simulink model "main_RI_LIEKF"  (R2023a)
settings: Solver=FixedStepAuto  StartTime=0.0  StopTime=220  FixedStep=0.01  RelTol=1e-3
InitFcn:
  | initNavigation0612_AOA;
values from neighbouring files (symbols this model uses):
  CF_enable = 0    [initNavigation.m]
  dt = 0.01    [initNavigation.m]
  dtDelay = -0.03    [initNavigation.m]
  g0 = 9.795    [initNavigation.m]
  gam0_rad = 0/57.3    (= 0)    [initNavigation.m]
  H_sensor_type = 0    [initNavigation.m]
  KF_enable = 1    [initNavigation.m]
  P0 = diag([1*ones(3,1);0.01*ones(3,1);0.1*ones(3,1);0.001*ones(3,1);0.00001*ones(3,1)])    [initNavigation.m]
  P0_RIEKF = diag([1*ones(3,1);0.01*ones(3,1);0.1*ones(3,1);0.001*ones(3,1);0.00001*ones(3,1);      0.01*ones(3,1);[0;2;2]/57.3;[0.1;0.1;0.1]])^2    [initNavigation.m]
  pd0 = 0    [initNavigation.m]
  pe0 = 0    [initNavigation.m]
  phi0_rad = 0/57.3    (= 0)    [initNavigation.m]
  pn0 = 0    [initNavigation.m]
  psi = -178    [initNavigation.m]
  psi0_rad = 0/57.3    (= 0)    [initNavigation.m]
  state_dim = 24    [initNavigation.m]
  Time = 0:0.01:(size(traindata.AttackAngle,1) - 1)*0.01    [NNLiftCoefficientFit.m]
  vd0 = 0    [initNavigation.m]
  ve0 = 0    [initNavigation.m]
  vn0 = 0    [initNavigation.m]
undefined symbols (not defined in the file or in its folder): DiscIntNeverNeededParam, Discrete, INS_CONST, INS_EXPORT, INS_PARAM, magnitude, p, param, pInitialization, sys
libraries: simulink x69, simulink_extras x64, dspstat3 x56, sharedtransform x49, ctrlSharedLib x36, sharedTrackingLibrary x17, FMT_Model_Lib x13, matrix_library x12, deeplib x4, dspsolvers x4, vrlib x4, aerolibconvert2 x1
(part 15 of 22)

== system main_RI_LIEKF/State estimation/bak1/INS propogation/Init_PVQ/Horizontal_attitude ==
  note: gamma
  note: fai
  accl_mean_B_m/s_LPF : Inport  PortDimensions=3
  Magn_mean_B_guess_LPF : Inport  Port=2
  Enable : EnablePort
  Add : Sum  Inputs=+-
  Asin : Trigonometry  Operator=asin
  Atan2 : Trigonometry  Operator=atan2
  Data Type Conversion : DataTypeConversion  SaturateOnIntegerOverflow=off  RndMeth=Floor
  Deal with zero : Subsystem
  Degrees to Radians : simulink_extras/Transformations/Degrees to Radians
  Degrees to Radians1 : simulink_extras/Transformations/Degrees to Radians
  Demux : Demux  Outputs=3
  Divide : Product  Inputs=*/  OutDataTypeStr=single
  Gain1 : Gain  Gain=-1
  Gain2 : Gain  Gain=-1
  Magnetic declination : Constant  Value=param.fusion.magDeclDeg  OutDataTypeStr=single
  Magnetic declination1 : Constant  Value=param.control.MagnheadingCorrection  OutDataTypeStr=uint8
  Math Function : Math  Operator=magnitude^2  SignedPower=on
  Mux : Mux  Inputs=3
  Mux1 : Mux  Inputs=3
  Mux3 : Mux  Inputs=3
  Product : Product  Multiplication=Matrix(*)
  Quaternions to Direction Cosine Matrix : sharedtransform/Quaternions to  Direction Cosine Matrix  aMode=aMode
  Rotation Angles to Quaternions : sharedtransform/Rotation Angles to Quaternions  rotationOrder=ZYX  aMode=aMode
  Rotation Angles to Quaternions1 : sharedtransform/Rotation Angles to Quaternions  rotationOrder=ZYX  aMode=aMode
  Scope : Scope
  Scope1 : Scope
  Selector : Selector  InputPortWidth=3  IndexOptions=Index vector (dialog)  Indices=[2]  OutputSizes=1
  Selector1 : Selector  InputPortWidth=3  IndexOptions=Index vector (dialog)  Indices=[1]  OutputSizes=1
  Sqrt : Sqrt
  Sum of Elements : Sum  Inputs=+
  Switch : Switch  Threshold=0.5  SaturateOnIntegerOverflow=off  InputSameDT=off
  Terminator : Terminator
  Transpose : Math  Operator=transpose  SignedPower=on
  Trigonometric Function1 : Trigonometry  Operator=atan2
  psi_zero : Constant  Value=psi  OutDataTypeStr=single
  quat_0 : Outport  PortDimensions=4
  wires:
  Data Type Conversion/1 -> Scope/1
  Switch/1 -> quat_0/1, Scope1/1
  Magnetic declination1/1 -> Switch/2, Data Type Conversion/1
  Degrees to Radians/1 -> Terminator/1
  Degrees to Radians1/1 -> Mux1/1
  Gain1/1 -> Mux/3, Trigonometric Function1/2
  Transpose/1 -> Product/1
  Mux3/1 -> Rotation Angles to Quaternions1/1
  Add/1 -> Mux3/1  "psi_calbymag"
  Magnetic declination/1 -> Degrees to Radians/1
  Atan2/1 -> Add/2
  Selector/1 -> Atan2/1  "magE"
  Selector1/1 -> Atan2/2  "magN"
  Product/1 -> Selector1/1, Selector/1  "magNED"
  Magn_mean_B_guess_LPF/1 -> Product/2
  Quaternions to Direction Cosine Matrix/1 -> Transpose/1
  Rotation Angles to Quaternions/1 -> Quaternions to Direction Cosine Matrix/1, Switch/3  "q0_no_yaw"
  Gain2/1 -> Mux1/3, Mux3/3
  Asin/1 -> Mux1/2, Mux3/2
  psi_zero/1 -> Degrees to Radians1/1
  Mux1/1 -> Rotation Angles to Quaternions/1
  Math Function/1 -> Sum of Elements/1
  Mux/1 -> Math Function/1
  Divide/1 -> Asin/1
  Sum of Elements/1 -> Sqrt/1
  Demux/3 -> Gain1/1
  Demux/2 -> Trigonometric Function1/1, Mux/1
  Demux/1 -> Mux/2, Divide/1
  Trigonometric Function1/1 -> Gain2/1
  Deal with zero/1(Out1) -> Divide/2
  Sqrt/1 -> Deal with zero/1(In1)
  accl_mean_B_m/s_LPF/1 -> Demux/1
  Rotation Angles to Quaternions1/1 -> Switch/1

== system main_RI_LIEKF/State estimation/bak1/INS propogation/Init_PVQ/Subsystem ==
  data : Inport
  Buffer : Buffer  N=50  V=49  OutputFrames=off
  Buffer1 : Buffer  N=50  V=49  OutputFrames=off
  Buffer2 : Buffer  N=50  V=49  ic=-g0  OutputFrames=off
  Demux : Demux  Outputs=3
  Mean4 : dspstat3/Mean  run=off  reset_popup=None  directionMode=Entire input  dimension=3  roiEnable=off  roiType=Rectangles  roiPortion=Entire ROI  roiOutput=Individual statistics for each ROI  roiFlag=off  roundingMode=Floor  overflowMode=off  outputDataTypeStr=Inherit: Same as accumulator  outputMin=[]  outputMax=[]  outputLastDataTypeStr=Inherit: Same as accumulator
  Mean5 : dspstat3/Mean  run=off  reset_popup=None  directionMode=Entire input  dimension=3  roiEnable=off  roiType=Rectangles  roiPortion=Entire ROI  roiOutput=Individual statistics for each ROI  roiFlag=off  roundingMode=Floor  overflowMode=off  outputDataTypeStr=Inherit: Same as accumulator  outputMin=[]  outputMax=[]  outputLastDataTypeStr=Inherit: Same as accumulator
  Mean6 : dspstat3/Mean  run=off  reset_popup=None  directionMode=Entire input  dimension=3  roiEnable=off  roiType=Rectangles  roiPortion=Entire ROI  roiOutput=Individual statistics for each ROI  roiFlag=off  roundingMode=Floor  overflowMode=off  outputDataTypeStr=Inherit: Same as accumulator  outputMin=[]  outputMax=[]  outputLastDataTypeStr=Inherit: Same as accumulator
  Scope : Scope  NumInputPorts=2
  Vector Concatenate : Concatenate  NumInputs=3
  mean_data : Outport
  wires:
  data/1 -> Demux/1, Scope/1
  Vector Concatenate/1 -> mean_data/1, Scope/2
  Mean4/1 -> Vector Concatenate/1
  Demux/3 -> Buffer2/1
  Buffer1/1 -> Mean5/1  "fby_buff"
  Demux/1 -> Buffer/1
  Buffer2/1 -> Mean6/1  "fbz_buff"
  Mean5/1 -> Vector Concatenate/2
  Buffer/1 -> Mean4/1  "fbx_buff"
  Demux/2 -> Buffer1/1
  Mean6/1 -> Vector Concatenate/3

== system main_RI_LIEKF/State estimation/bak1/INS propogation/Init_PVQ/Subsystem1 ==
  data : Inport
  Buffer : Buffer  N=50  V=49  OutputFrames=off
  Buffer1 : Buffer  N=50  V=49  OutputFrames=off
  Buffer2 : Buffer  N=50  V=49  OutputFrames=off
  Demux : Demux  Outputs=3
  Mean4 : dspstat3/Mean  run=off  reset_popup=None  directionMode=Entire input  dimension=3  roiEnable=off  roiType=Rectangles  roiPortion=Entire ROI  roiOutput=Individual statistics for each ROI  roiFlag=off  roundingMode=Floor  overflowMode=off  outputDataTypeStr=Inherit: Same as accumulator  outputMin=[]  outputMax=[]  outputLastDataTypeStr=Inherit: Same as accumulator
  Mean5 : dspstat3/Mean  run=off  reset_popup=None  directionMode=Entire input  dimension=3  roiEnable=off  roiType=Rectangles  roiPortion=Entire ROI  roiOutput=Individual statistics for each ROI  roiFlag=off  roundingMode=Floor  overflowMode=off  outputDataTypeStr=Inherit: Same as accumulator  outputMin=[]  outputMax=[]  outputLastDataTypeStr=Inherit: Same as accumulator
  Mean6 : dspstat3/Mean  run=off  reset_popup=None  directionMode=Entire input  dimension=3  roiEnable=off  roiType=Rectangles  roiPortion=Entire ROI  roiOutput=Individual statistics for each ROI  roiFlag=off  roundingMode=Floor  overflowMode=off  outputDataTypeStr=Inherit: Same as accumulator  outputMin=[]  outputMax=[]  outputLastDataTypeStr=Inherit: Same as accumulator
  Vector Concatenate : Concatenate  NumInputs=3
  mean_data : Outport
  wires:
  Mean6/1 -> Vector Concatenate/3
  Demux/2 -> Buffer1/1
  Buffer/1 -> Mean4/1  "fbx_buff"
  Mean5/1 -> Vector Concatenate/2
  Buffer2/1 -> Mean6/1  "fbz_buff"
  Demux/1 -> Buffer/1
  Buffer1/1 -> Mean5/1  "fby_buff"
  Demux/3 -> Buffer2/1
  Mean4/1 -> Vector Concatenate/1
  Vector Concatenate/1 -> mean_data/1
  data/1 -> Demux/1

== system main_RI_LIEKF/State estimation/bak1/INS propogation/accl bias compensation/error compensation1 ==
  dda : Inport
  Add3 : Sum
  Memory1 : Memory
  da : Outport
  wires:
  dda/1 -> Add3/1
  Memory1/1 -> Add3/2
  Add3/1 -> Memory1/1, da/1

== system main_RI_LIEKF/State estimation/bak1/INS propogation/gyro bias compensation/error compensation ==
  ddg : Inport
  Enable : Inport  Port=2
  Add3 : Sum
  Data Store Read5 : DataStoreRead  DataStoreName=GPS_enable  IndexOptions=Index vector (dialog)  Indices=1  OutputSizes=1
  If Action Subsystem1 : Subsystem  TreatAsAtomicUnit=on
  If1 : If  IfExpression=u1 == 1  ShowElse=off
  Memory1 : Memory
  Scope : Scope
  dg : Outport
  wires:
  ddg/1 -> Add3/1
  Add3/1 -> Memory1/1, dg/1
  Memory1/1 -> Add3/2
  If1/1 -> If Action Subsystem1/Action
  Enable/1 -> If1/1, Scope/1

== system main_RI_LIEKF/State estimation/bak1/INS propogation/vel_pos_update/Kinematic Equation ==
  Cbn : Inport
  Ab : Inport  Port=2
  Add : Sum  Inputs=+-
  Constant : Constant  Value=[0 0 -g0]  OutDataTypeStr=single
  Product : Product  Multiplication=Matrix(*)  RndMeth=Zero
  Scope : Scope
  Scope1 : Scope  NumInputPorts=2
  An : Outport
  wires:
  Constant/1 -> Add/2
  Product/1 -> Add/1, Scope/1
  Ab/1 -> Scope1/1, Product/2
  Add/1 -> Scope1/2, An/1
  Cbn/1 -> Product/1

== system main_RI_LIEKF/State estimation/bak1/INS propogation/vel_pos_update/pos update ==
  dtheta : Inport
  vel_k : Inport  Port=2
  dp : Inport  Port=3
  QGC_init : Inport  Port=4
  p0 : Inport  Port=5
  Add1 : Sum
  Delay1 : Delay  DelayLength=1  InitialConditionSource=Input port  ExternalReset=Rising
      settings: InputPortMap=u0,r5,p4
  Gain1 : Gain  Gain=dt
  MATLAB Function : MATLAB Function  TreatAsAtomicUnit=on
  Reshape1 : Reshape  OutputDimensionality=Column vector (2-D)
  p_k : Outport
  wires:
  MATLAB Function/1(pos_correct) -> p_k/1, Delay1/1
  Add1/1 -> MATLAB Function/3(pos)
  dp/1 -> MATLAB Function/2(KFState_dp)
  dtheta/1 -> MATLAB Function/1(dtheta)
  vel_k/1 -> Gain1/1
  Gain1/1 -> Add1/1
  Delay1/1 -> Add1/2
  Reshape1/1 -> Delay1/3
  QGC_init/1 -> Delay1/2
  p0/1 -> Reshape1/1

== system main_RI_LIEKF/State estimation/bak1/INS propogation/vel_pos_update/vel update ==
  dtheta : Inport
  QGC_init : Inport  Port=2
  An : Inport  Port=3
  KFState_dv : Inport  Port=4
  v0 : Inport  Port=5
  Add : Sum
  Delay : Delay  DelayLength=1  InitialConditionSource=Input port  ExternalReset=Rising
      settings: InputPortMap=u0,r5,p4
  Gain : Gain  Gain=dt
  MATLAB Function : MATLAB Function  TreatAsAtomicUnit=on
  Reshape : Reshape  OutputDimensionality=Column vector (2-D)
  vel_k : Outport
  wires:
  MATLAB Function/1(vel_correct) -> vel_k/1, Delay/1
  Add/1 -> MATLAB Function/3(vel)
  dtheta/1 -> MATLAB Function/1(dtheta)
  KFState_dv/1 -> MATLAB Function/2(KFState_dv)
  Delay/1 -> Add/2
  Gain/1 -> Add/1
  v0/1 -> Reshape/1
  An/1 -> Gain/1
  Reshape/1 -> Delay/3
  QGC_init/1 -> Delay/2

== system main_RI_LIEKF/State estimation/distribute CF/AHRS/AHRS Complementary filter/Complementary Filter ==
  note: 1：匀速运动或静止状态
      | 2：加速运动有GPS
      | 3：加速运动没GPS
  fbxyz : Inport
  Fly_status : Inport  Port=2
  fb_estimatedValue : Inport  Port=3
  Cross-product : Subsystem
      mask DialogControl Control2 Prompt: Vector A×B
  Discrete-Time Integrator1 : DiscreteIntegrator  SampleTime=-1  LimitOutput=on  UpperSaturationLimit=0.005  LowerSaturationLimit=-0.005  ICPrevOutput=DiscIntNeverNeededParam  ICPrevScaledInput=DiscIntNeverNeededParam
  Discrete-Time Integrator2 : DiscreteIntegrator  SampleTime=-1  LimitOutput=on  UpperSaturationLimit=0.005  LowerSaturationLimit=-0.005  ICPrevOutput=DiscIntNeverNeededParam  ICPrevScaledInput=DiscIntNeverNeededParam
  Gain : Gain  Gain=GPS_accel_kp
  Gain2 : Gain  Gain=noGPS_accel_kp
  Gain3 : Gain  Gain=GPS_accel_ki
  Gain4 : Gain  Gain=noGPS_accel_ki
  Normalized : Subsystem
  Normalized1 : Subsystem
  Scope : Scope
  Scope1 : Scope
  Scope2 : Scope
  Sum : Sum  Inputs=|++
  Sum1 : Sum  Inputs=|++
  Switch : Switch  Threshold=2  SaturateOnIntegerOverflow=off  InputSameDT=off
  w_bias : Outport
  wires:
  Discrete-Time Integrator2/1 -> Sum/2
  Discrete-Time Integrator1/1 -> Sum1/2
  Cross-product/1(vactor_error_A&B) -> Gain/1, Gain3/1, Gain4/1, Gain2/1, Scope1/1
  Normalized/1(fb/g) -> Cross-product/1(vactor_A)
  Normalized1/1(fb_estimatedValue_Normalized) -> Cross-product/2(vactor_B), Scope2/1
  Sum/1 -> Switch/3
  Sum1/1 -> Switch/1
  Switch/1 -> w_bias/1, Scope/1
  Gain4/1 -> Discrete-Time Integrator1/1
  Gain2/1 -> Sum1/1
  Gain3/1 -> Discrete-Time Integrator2/1
  Gain/1 -> Sum/1
  Fly_status/1 -> Switch/2
  fb_estimatedValue/1 -> Normalized1/1(fb_estimatedValue)
  fbxyz/1 -> Normalized/1(fb)

== system main_RI_LIEKF/State estimation/distribute CF/AHRS/AHRS Complementary filter/GPSHeadingCorrect ==
  GPSdata : Inport
  Q_update : Inport  Port=2
  Add : Sum  Inputs=+-
  Bus Selector3 : BusSelector  OutputSignals=q_update
  Bus Selector4 : BusSelector  OutputSignals=heading_GPS_rad,heading_GPS_valid
  Constant : Constant  Value=0
  Constant1 : Constant  Value=0
  Data Type Conversion : DataTypeConversion  OutDataTypeStr=double  SaturateOnIntegerOverflow=off  RndMeth=Floor
  Data Type Conversion1 : DataTypeConversion  OutDataTypeStr=single  SaturateOnIntegerOverflow=off  RndMeth=Floor
  Data Type Conversion2 : DataTypeConversion  OutDataTypeStr=double  SaturateOnIntegerOverflow=off  RndMeth=Floor
  Discrete-Time Integrator : DiscreteIntegrator  SampleTime=-1  ICPrevOutput=DiscIntNeverNeededParam  ICPrevScaledInput=DiscIntNeverNeededParam
  Gain : Gain  Gain=0.2
  Gain1 : Gain  Gain=0
  Gain2 : Gain  Gain=param.control.GPSheadingCorrection
  Mux : Mux  Inputs=2
  Mux2 : Mux  Inputs=3
  Quaternions to Rotation Angles : sharedtransform/Quaternions to Rotation Angles  rotationOrder=ZYX  aMode=aMode
  Selector : Selector  InputPortWidth=3  IndexOptions=Index vector (dialog)  Indices=[2 3]  OutputSizes=1
  Selector1 : Selector  InputPortWidth=3  IndexOptions=Index vector (dialog)  Indices=[1]  OutputSizes=1
  Sum : Sum  Inputs=|++
  Switch : Switch  Threshold=1  SaturateOnIntegerOverflow=off  InputSameDT=off
  wz_bias_by_GPS : Outport
  PsiGPS&pitch&roll : Outport  Port=2
  wires:
  GPSdata/1 -> Bus Selector4/1
  Mux/1 -> PsiGPS&pitch&roll/1
  Selector1/1 -> Add/1
  Data Type Conversion1/1 -> Gain2/1
  Constant/1 -> Mux2/1, Mux2/2
  Bus Selector4/2 -> Switch/2  "<heading_GPS_valid>"
  Data Type Conversion2/1 -> Mux/1, Add/2
  Constant1/1 -> Switch/3
  Add/1 -> Mux2/3
  Mux2/1 -> Gain1/1, Gain/1
  Gain2/1 -> wz_bias_by_GPS/1
  Switch/1 -> Data Type Conversion1/1
  Data Type Conversion/1 -> Quaternions to Rotation Angles/1
  Q_update/1 -> Bus Selector3/1
  Selector/1 -> Mux/2
  Quaternions to Rotation Angles/1 -> Selector/1, Selector1/1
  Bus Selector4/1 -> Data Type Conversion2/1  "<heading_GPS_rad>"
  Bus Selector3/1 -> Data Type Conversion/1  "<q_update>"
  Gain/1 -> Sum/1
  Sum/1 -> Switch/1
  Discrete-Time Integrator/1 -> Sum/2
  Gain1/1 -> Discrete-Time Integrator/1

== system main_RI_LIEKF/State estimation/distribute CF/AHRS/AHRS Complementary filter/MagnHeadingCorrect ==
  Cbn : Inport
  Magnxyz : Inport  Port=2
  Constant5 : Constant  Value=0  OutDataTypeStr=single
  Discrete-Time Integrator1 : DiscreteIntegrator  gainval=1  SampleTime=-1  ICPrevOutput=DiscIntNeverNeededParam  ICPrevScaledInput=DiscIntNeverNeededParam
  Fcn1 : Fcn  Expr=u(3)
  Fcn2 : Fcn  Expr=sqrt(u(1)*u(1)+u(2)*u(2))
  Gain11 : Gain  Gain=0.2
  Gain12 : Gain  Gain=[0;0;1]
  Gain14 : Gain  Gain=0
  Gain2 : Gain  Gain=param.control.MagnheadingCorrection
  Math Function4 : Math  Operator=transpose  SignedPower=on
  Mux1 : Mux  Inputs=3
  Product3 : Product  Multiplication=Matrix(*)  SaturateOnIntegerOverflow=on  OutDataTypeStr=Inherit: Same as first input
  Product6 : Product  Multiplication=Matrix(*)  SaturateOnIntegerOverflow=on  OutDataTypeStr=Inherit: Same as first input
  Subsystem6 : Subsystem
  Sum4 : Sum  Inputs=|++
  chacheng6 : Subsystem
  wz_bias_by_magn : Outport
  wires:
  Subsystem6/1(m/|m|) -> Product3/2, chacheng6/2(In2)
  Product6/1 -> chacheng6/1(In1)
  Gain2/1 -> wz_bias_by_magn/1
  Cbn/1 -> Math Function4/1, Product3/1
  Fcn2/1 -> Mux1/1
  Constant5/1 -> Mux1/2
  Mux1/1 -> Product6/2
  Math Function4/1 -> Product6/1
  Gain12/1 -> Gain14/1, Gain11/1
  Gain11/1 -> Sum4/1
  Magnxyz/1 -> Subsystem6/1(m)
  chacheng6/1(Out1) -> Gain12/1
  Product3/1 -> Fcn2/1, Fcn1/1
  Fcn1/1 -> Mux1/3
  Discrete-Time Integrator1/1 -> Sum4/2
  Gain14/1 -> Discrete-Time Integrator1/1
  Sum4/1 -> Gain2/1

== system main_RI_LIEKF/State estimation/distribute CF/AHRS/AHRS Complementary filter/Trace differentiator ==
  originalVariable : Inport
  Constant1 : Constant  Value=0.01  OutDataTypeStr=single
  Constant2 : Constant  Value=0.01  OutDataTypeStr=single
  Constant3 : Constant  Value=0.2  OutDataTypeStr=single
  Constant4 : Constant  Value=900  OutDataTypeStr=single
  Constant5 : Constant  Value=0.2  OutDataTypeStr=single
  Constant6 : Constant  Value=900  OutDataTypeStr=single
  Constant7 : Constant  Value=0.01  OutDataTypeStr=single
  Constant8 : Constant  Value=0.2  OutDataTypeStr=single
  Constant9 : Constant  Value=900  OutDataTypeStr=single
  Demux : Demux  Outputs=3
  MATLAB Function1 : MATLAB Function  TreatAsAtomicUnit=on
  MATLAB Function2 : MATLAB Function  TreatAsAtomicUnit=on
  MATLAB Function3 : MATLAB Function  TreatAsAtomicUnit=on
  Memory{,1..5} (6 alike) : Memory  InheritSampleTime=on
  Mux : Mux  Inputs=3
  originalVariableDifference : Outport
  wires:
  MATLAB Function2/1(u1) -> Memory/1
  Constant4/1 -> MATLAB Function2/6(r)
  Constant1/1 -> MATLAB Function2/1(T)
  Constant3/1 -> MATLAB Function2/5(h)
  MATLAB Function2/2(u2) -> Memory1/1
  Memory/1 -> MATLAB Function2/3("u1 ")
  Memory1/1 -> Mux/1, MATLAB Function2/4("u2 ")
  Memory3/1 -> MATLAB Function1/4("u2 "), Mux/2
  Memory2/1 -> MATLAB Function1/3("u1 ")
  MATLAB Function1/2(u2) -> Memory3/1
  Constant5/1 -> MATLAB Function1/5(h)
  Constant2/1 -> MATLAB Function1/1(T)
  Constant6/1 -> MATLAB Function1/6(r)
  MATLAB Function1/1(u1) -> Memory2/1
  MATLAB Function3/1(u1) -> Memory4/1
  Constant9/1 -> MATLAB Function3/6(r)
  Constant7/1 -> MATLAB Function3/1(T)
  Constant8/1 -> MATLAB Function3/5(h)
  MATLAB Function3/2(u2) -> Memory5/1
  Memory4/1 -> MATLAB Function3/3("u1 ")
  Memory5/1 -> Mux/3, MATLAB Function3/4("u2 ")
  Mux/1 -> originalVariableDifference/1
  originalVariable/1 -> Demux/1
  Demux/1 -> MATLAB Function2/2(u0)
  Demux/2 -> MATLAB Function1/2(u0)
  Demux/3 -> MATLAB Function3/2(u0)

== system main_RI_LIEKF/State estimation/distribute CF/AHRS/AHRS Complementary filter/UAV_accelerate_within_gravity_estimate ==
  note: 1：匀速运动或静止状态
      | 2：加速运动有GPS
      | 3：加速运动没GPS
  Fly_status : Inport
  GPS_type : Inport  Port=2
  <DCM_b_n> : Inport  Port=3
  accel_GPS_ned : Inport  Port=4
  Add2 : Sum
  Compare To Zero : simulink/Logic and Bit Operations/Compare To Zero  relop===  OutDataTypeStr=boolean
  Constant : Constant  Value=[0;0;-1]
  Constant1 : Constant  Value=[0;0;0]  OutDataTypeStr=single
  Gain2 : Gain  Gain=g0
  Logical Operator : Logic  Operator=NOT  AllPortsSameDT=off  OutDataTypeStr=boolean
  Math Function1 : Math  Operator=transpose  SignedPower=on
  Memory : Memory
  Multiport Switch : MultiPortSwitch  Inputs=2  DataPortForDefault=Additional data port  DiagnosticForDefault=None  SaturateOnIntegerOverflow=off  InputSameDT=off
  Product : Product  Multiplication=Matrix(*)  SaturateOnIntegerOverflow=on  OutDataTypeStr=Inherit: Same as first input
  Product1 : Product  Multiplication=Matrix(*)  SaturateOnIntegerOverflow=on  OutDataTypeStr=Inherit: Same as first input
  Product2 : Product
  Scope : Scope
  Scope1 : Scope
  Scope2 : Scope
  accelerate_within_gravity_estimate : Outport
  wires:
  Product1/1 -> Add2/1
  Fly_status/1 -> Scope2/1, Multiport Switch/1
  Memory/1 -> Product2/2
  Product2/1 -> Scope1/1
  Logical Operator/1 -> Memory/1
  Compare To Zero/1 -> Logical Operator/1
  GPS_type/1 -> Compare To Zero/1, Scope/1
  Add2/1 -> Product2/1
  Multiport Switch/1 -> accelerate_within_gravity_estimate/1
  Gain2/1 -> Add2/2, Multiport Switch/2, Multiport Switch/4
  Constant/1 -> Product/2
  Product/1 -> Gain2/1
  accel_GPS_ned/1 -> Product1/2  "accel_GPS_ned"
  Math Function1/1 -> Product/1, Product1/1  "DCM_n_b"
  <DCM_b_n>/1 -> Math Function1/1

== system main_RI_LIEKF/State estimation/distribute CF/AHRS/AHRS Complementary filter/gyro_preprocessing2 ==
  note: rad/s
  note: front-right-dowm
  gyro_B_rad/s_ori : Inport
  Constant2 : Constant  Value=1/dt  OutDataTypeStr=single
  Constant4 : Constant  Value=1/dt  OutDataTypeStr=single
  Constant6 : Constant  Value=1/dt  OutDataTypeStr=single
  Constant7 : Constant  Value=30  OutDataTypeStr=single
  Demux : Demux  Outputs=3
  MATLAB Function1 : MATLAB Function  TreatAsAtomicUnit=on
  MATLAB Function2 : MATLAB Function  TreatAsAtomicUnit=on
  MATLAB Function3 : MATLAB Function  TreatAsAtomicUnit=on
  Scope : Scope  NumInputPorts=2
  Vector Concatenate : Concatenate  NumInputs=3
  gyro_B_rad/s_LPF : Outport  PortDimensions=3
  wires:
  Vector Concatenate/1 -> Scope/1, gyro_B_rad/s_LPF/1
  Constant4/1 -> MATLAB Function2/2(sample_freq)
  Constant2/1 -> MATLAB Function1/2(sample_freq)
  gyro_B_rad/s_ori/1 -> Scope/2, Demux/1
  Demux/1 -> MATLAB Function2/1(curr_input)
  Demux/2 -> MATLAB Function1/1(curr_input)
  Constant6/1 -> MATLAB Function3/2(sample_freq)
  Demux/3 -> MATLAB Function3/1(curr_input)
  Constant7/1 -> MATLAB Function2/3(cutoff_freq), MATLAB Function1/3(cutoff_freq), MATLAB Function3/3(cutoff_freq)
  MATLAB Function3/1(curr_output) -> Vector Concatenate/3  "wz"
  MATLAB Function1/1(curr_output) -> Vector Concatenate/2  "wy"
  MATLAB Function2/1(curr_output) -> Vector Concatenate/1  "wx"

== system main_RI_LIEKF/State estimation/distribute CF/AHRS/AHRS Complementary filter/manoeuvrable check ==
  note: 1：匀速运动或静止状态
      | 2：加速运动有GPS
      | 3：加速运动没GPS
  accel_GPS_ned : Inport
  fbxyz1 : Inport  Port=2
  DCM_b_n : Inport  Port=3
  fixtype_GPS : Inport  Port=4
  Compare To Constant1 : simulink/Logic and Bit Operations/Compare To Constant  relop=>=  const=0.1  OutDataTypeStr=boolean
  Compare To Constant2 : simulink/Logic and Bit Operations/Compare To Constant  relop=>=  const=1  OutDataTypeStr=boolean
  Constant1 : Constant  Value=3  OutDataTypeStr=uint8
  Constant3 : Constant  Value=2  OutDataTypeStr=uint8
  Constant4 : Constant  OutDataTypeStr=uint8
  Data Type Conversion : DataTypeConversion  OutDataTypeStr=double  SaturateOnIntegerOverflow=off  RndMeth=Floor
  Direction Cosine Matrix to Rotation Angles : sharedtransform/Direction Cosine Matrix to Rotation Angles  rotationOrder=ZYX  aMode=aMode  action=None  tolerance=eps(2)
  Display : Display
  Display1 : Display
  Display2 : Display
  Logical Operator1 : Logic  AllPortsSameDT=off  OutDataTypeStr=boolean
  Logical Operator2 : Logic  Operator=NOT  AllPortsSameDT=off  OutDataTypeStr=boolean
  Logical Operator3 : Logic  AllPortsSameDT=off  OutDataTypeStr=boolean
  Logical Operator4 : Logic  AllPortsSameDT=off  OutDataTypeStr=boolean
  Math Function : Math  Operator=magnitude^2  SignedPower=on
  Product : Product  Multiplication=Matrix(*)
  Scope{,1..3} (4 alike) : Scope
  Scope4 : Scope  NumInputPorts=2
  Sqrt : Sqrt
  Sum of Elements : Sum  Inputs=+
  Switch1 : Switch  Threshold=1  SaturateOnIntegerOverflow=off  InputSameDT=off
  Switch2 : Switch  Threshold=1  SaturateOnIntegerOverflow=off  InputSameDT=off
  Transpose : Math  Operator=transpose  SignedPower=on
  manoeuvrable check : Subsystem
      mask DialogControl DescTextVar Prompt: manoeuvrable check
      mask DialogControl Control2 Prompt: flag = 0 : 机动状态
      mask DialogControl Control3 Prompt: flag = 1：静止/匀速状态
  Fly_status : Outport
  wires:
  Data Type Conversion/1 -> Direction Cosine Matrix to Rotation Angles/1
  Transpose/1 -> Data Type Conversion/1
  Direction Cosine Matrix to Rotation Angles/1 -> manoeuvrable check/2(eular)
  Switch2/1 -> Fly_status/1, Scope/1, Display2/1
  Switch1/1 -> Switch2/3
  Constant4/1 -> Switch1/3
  Constant1/1 -> Switch1/1
  Logical Operator3/1 -> Switch1/2
  Logical Operator2/1 -> Logical Operator3/2, Display/1, Scope3/1
  Constant3/1 -> Switch2/1
  Logical Operator1/1 -> Switch2/2
  Compare To Constant2/1 -> Scope4/1
  manoeuvrable check/1(flag) -> Logical Operator1/2, Logical Operator3/1, Display1/1, Scope1/1
  fixtype_GPS/1 -> Compare To Constant2/1
  Compare To Constant1/1 -> Scope4/2
  Sqrt/1 -> Compare To Constant1/1
  Sum of Elements/1 -> Sqrt/1
  Product/1 -> manoeuvrable check/1(fn), Scope2/1
  DCM_b_n/1 -> Product/1, Transpose/1
  fbxyz1/1 -> Product/2
  Math Function/1 -> Sum of Elements/1
  accel_GPS_ned/1 -> Math Function/1

== system main_RI_LIEKF/State estimation/distribute CF/AHRS/Init_Q0/Horizontal_attitude ==
  note: gamma
  note: fai
  accl_mean_B_m/s_LPF : Inport  PortDimensions=3
  Magn_mean_B_guess_LPF : Inport  Port=2
  Enable : EnablePort
  Add : Sum  Inputs=+-
  Add1 : Sum
  Add2 : Sum
  Add3 : Sum
  Asin : Trigonometry  Operator=asin
  Atan2 : Trigonometry  Operator=atan2
  Data Type Conversion : DataTypeConversion  SaturateOnIntegerOverflow=off  RndMeth=Floor
  Deal with zero : Subsystem
  Degrees to Radians : simulink_extras/Transformations/Degrees to Radians
  Degrees to Radians1 : simulink_extras/Transformations/Degrees to Radians
  Demux : Demux  Outputs=3
  Divide : Product  Inputs=*/  OutDataTypeStr=single
  Gain1 : Gain  Gain=-1
  Gain2 : Gain  Gain=-1
  Magnetic declination : Constant  Value=param.fusion.magDeclDeg  OutDataTypeStr=single
  Magnetic declination1 : Constant  Value=param.control.MagnheadingCorrection  OutDataTypeStr=uint8
  Math Function : Math  Operator=magnitude^2  SignedPower=on
  Mux : Mux  Inputs=3
  Mux1 : Mux  Inputs=3
  Mux3 : Mux  Inputs=3
  Product : Product  Multiplication=Matrix(*)
  Quaternions to Direction Cosine Matrix : sharedtransform/Quaternions to  Direction Cosine Matrix  aMode=aMode
  Rotation Angles to Quaternions : sharedtransform/Rotation Angles to Quaternions  rotationOrder=ZYX  aMode=aMode
  Rotation Angles to Quaternions1 : sharedtransform/Rotation Angles to Quaternions  rotationOrder=ZYX  aMode=aMode
  Scope : Scope
  Scope1 : Scope
  Selector : Selector  InputPortWidth=3  IndexOptions=Index vector (dialog)  Indices=[2]  OutputSizes=1
  Selector1 : Selector  InputPortWidth=3  IndexOptions=Index vector (dialog)  Indices=[1]  OutputSizes=1
  Sqrt : Sqrt
  Sum of Elements : Sum  Inputs=+
  Switch : Switch  Threshold=0.5  SaturateOnIntegerOverflow=off  InputSameDT=off
  Terminator : Terminator
  Transpose : Math  Operator=transpose  SignedPower=on
  Trigonometric Function1 : Trigonometry  Operator=atan2
  psi_zero : Constant  Value=psi  OutDataTypeStr=single
  psi_zero1 : Constant  Value=psi0_rad  OutDataTypeStr=single
  psi_zero2 : Constant  Value=phi0_rad  OutDataTypeStr=single
  psi_zero3 : Constant  Value=gam0_rad  OutDataTypeStr=single
  quat_0 : Outport  PortDimensions=4
  wires:
  Data Type Conversion/1 -> Scope/1
  Rotation Angles to Quaternions1/1 -> Switch/1
  Switch/1 -> quat_0/1, Scope1/1
  Magnetic declination1/1 -> Switch/2, Data Type Conversion/1
  Degrees to Radians/1 -> Terminator/1
  Add1/1 -> Mux1/1
  Gain1/1 -> Mux/3, Trigonometric Function1/2
  Transpose/1 -> Product/1
  Mux3/1 -> Rotation Angles to Quaternions1/1
  Add/1 -> Mux3/1  "psi_calbymag"
  Magnetic declination/1 -> Degrees to Radians/1
  Atan2/1 -> Add/2
  Selector/1 -> Atan2/1  "magE"
  Selector1/1 -> Atan2/2  "magN"
  Product/1 -> Selector1/1, Selector/1  "magNED"
  Magn_mean_B_guess_LPF/1 -> Product/2
  Quaternions to Direction Cosine Matrix/1 -> Transpose/1
  Rotation Angles to Quaternions/1 -> Quaternions to Direction Cosine Matrix/1, Switch/3  "q0_no_yaw"
  Add3/1 -> Mux3/3, Mux1/3
  Add2/1 -> Mux1/2, Mux3/2
  psi_zero/1 -> Degrees to Radians1/1
  Mux1/1 -> Rotation Angles to Quaternions/1
  Math Function/1 -> Sum of Elements/1
  Mux/1 -> Math Function/1
  Divide/1 -> Asin/1
  Sum of Elements/1 -> Sqrt/1
  Demux/3 -> Gain1/1
  Demux/2 -> Trigonometric Function1/1, Mux/1
  Demux/1 -> Mux/2, Divide/1
  Trigonometric Function1/1 -> Gain2/1
  Deal with zero/1(Out1) -> Divide/2
  Sqrt/1 -> Deal with zero/1(In1)
  accl_mean_B_m/s_LPF/1 -> Demux/1
  psi_zero1/1 -> ?
  Degrees to Radians1/1 -> Add1/2
  psi_zero2/1 -> ?
  Asin/1 -> Add2/2
  psi_zero3/1 -> ?
  Gain2/1 -> Add3/2

== system main_RI_LIEKF/State estimation/distribute CF/AHRS/Init_Q0/Subsystem ==
  data : Inport
  Buffer : Buffer  N=50  V=49  OutputFrames=off
  Buffer1 : Buffer  N=50  V=49  OutputFrames=off
  Buffer2 : Buffer  N=50  V=49  ic=-g0  OutputFrames=off
  Demux : Demux  Outputs=3
  Mean4 : dspstat3/Mean  run=off  reset_popup=None  directionMode=Entire input  dimension=3  roiEnable=off  roiType=Rectangles  roiPortion=Entire ROI  roiOutput=Individual statistics for each ROI  roiFlag=off  roundingMode=Floor  overflowMode=off  outputDataTypeStr=Inherit: Same as accumulator  outputMin=[]  outputMax=[]  outputLastDataTypeStr=Inherit: Same as accumulator
  Mean5 : dspstat3/Mean  run=off  reset_popup=None  directionMode=Entire input  dimension=3  roiEnable=off  roiType=Rectangles  roiPortion=Entire ROI  roiOutput=Individual statistics for each ROI  roiFlag=off  roundingMode=Floor  overflowMode=off  outputDataTypeStr=Inherit: Same as accumulator  outputMin=[]  outputMax=[]  outputLastDataTypeStr=Inherit: Same as accumulator
  Mean6 : dspstat3/Mean  run=off  reset_popup=None  directionMode=Entire input  dimension=3  roiEnable=off  roiType=Rectangles  roiPortion=Entire ROI  roiOutput=Individual statistics for each ROI  roiFlag=off  roundingMode=Floor  overflowMode=off  outputDataTypeStr=Inherit: Same as accumulator  outputMin=[]  outputMax=[]  outputLastDataTypeStr=Inherit: Same as accumulator
  Scope : Scope  NumInputPorts=2
  Vector Concatenate : Concatenate  NumInputs=3
  mean_data : Outport
  wires:
  data/1 -> Demux/1, Scope/1
  Vector Concatenate/1 -> mean_data/1, Scope/2
  Mean4/1 -> Vector Concatenate/1
  Demux/3 -> Buffer2/1
  Buffer1/1 -> Mean5/1  "fby_buff"
  Demux/1 -> Buffer/1
  Buffer2/1 -> Mean6/1  "fbz_buff"
  Mean5/1 -> Vector Concatenate/2
  Buffer/1 -> Mean4/1  "fbx_buff"
  Demux/2 -> Buffer1/1
  Mean6/1 -> Vector Concatenate/3

== system main_RI_LIEKF/State estimation/distribute CF/AHRS/Init_Q0/Subsystem1 ==
  data : Inport
  Buffer : Buffer  N=50  V=49  OutputFrames=off
  Buffer1 : Buffer  N=50  V=49  OutputFrames=off
  Buffer2 : Buffer  N=50  V=49  OutputFrames=off
  Demux : Demux  Outputs=3
  Mean4 : dspstat3/Mean  run=off  reset_popup=None  directionMode=Entire input  dimension=3  roiEnable=off  roiType=Rectangles  roiPortion=Entire ROI  roiOutput=Individual statistics for each ROI  roiFlag=off  roundingMode=Floor  overflowMode=off  outputDataTypeStr=Inherit: Same as accumulator  outputMin=[]  outputMax=[]  outputLastDataTypeStr=Inherit: Same as accumulator
  Mean5 : dspstat3/Mean  run=off  reset_popup=None  directionMode=Entire input  dimension=3  roiEnable=off  roiType=Rectangles  roiPortion=Entire ROI  roiOutput=Individual statistics for each ROI  roiFlag=off  roundingMode=Floor  overflowMode=off  outputDataTypeStr=Inherit: Same as accumulator  outputMin=[]  outputMax=[]  outputLastDataTypeStr=Inherit: Same as accumulator
  Mean6 : dspstat3/Mean  run=off  reset_popup=None  directionMode=Entire input  dimension=3  roiEnable=off  roiType=Rectangles  roiPortion=Entire ROI  roiOutput=Individual statistics for each ROI  roiFlag=off  roundingMode=Floor  overflowMode=off  outputDataTypeStr=Inherit: Same as accumulator  outputMin=[]  outputMax=[]  outputLastDataTypeStr=Inherit: Same as accumulator
  Vector Concatenate : Concatenate  NumInputs=3
  mean_data : Outport
  wires:
  Mean6/1 -> Vector Concatenate/3
  Demux/2 -> Buffer1/1
  Buffer/1 -> Mean4/1  "fbx_buff"
  Mean5/1 -> Vector Concatenate/2
  Buffer2/1 -> Mean6/1  "fbz_buff"
  Demux/1 -> Buffer/1
  Buffer1/1 -> Mean5/1  "fby_buff"
  Demux/3 -> Buffer2/1
  Mean4/1 -> Vector Concatenate/1
  Vector Concatenate/1 -> mean_data/1
  data/1 -> Demux/1

== system main_RI_LIEKF/State estimation/distribute CF/AHRS/att_update/uniformization ==
  Q i : Inport  PortDimensions=4
  Constant : Constant  Value=1e-20
  Dot Product1 : DotProduct  OutDataTypeStr=Inherit: Inherit via internal rule
  Math Function : Math  Operator=sqrt  SignedPower=on
  Product : Product  Inputs=*/  SaturateOnIntegerOverflow=on  OutDataTypeStr=Inherit: Same as first input
  Sum : Sum  Inputs=|++  SaturateOnIntegerOverflow=on
  Q o : Outport
  wires:
  Sum/1 -> Product/2
  Constant/1 -> Sum/2
  Product/1 -> Q o/1
  Math Function/1 -> Sum/1
  Dot Product1/1 -> Math Function/1
  Q i/1 -> Product/1, Dot Product1/1, Dot Product1/2

== system main_RI_LIEKF/State estimation/distribute CF/Translation_estimate/Rxy_Horizontal_estimation/Integrator_R_Horizontal ==
  Vn : Inport
  dR : Inport  Port=2
  Sensor_data2 : Inport  Port=3
  Bus Selector : BusSelector  OutputSignals=QGC_sensor_reinit,GPS_Data.pos_N_gps,GPS_Data.pos_E_gps
  Delay : Delay  DelayLength=1  InitialConditionSource=Input port  ExternalReset=Rising
      settings: InputPortMap=u0,r5,p4
  Gain : Gain  Gain=0.8
  Gain2 : Gain  Gain=dt  SaturateOnIntegerOverflow=on  OutDataTypeStr=Inherit: Same as input  ParamDataTypeStr=Inherit: Same as input
  Mux : Mux  Inputs=2
  Sum : Sum  Inputs=|++-
  R_n&e : Outport
  wires:
  Gain/1 -> Sum/3
  dR/1 -> Gain/1
  Vn/1 -> Gain2/1
  Gain2/1 -> Sum/1
  Sum/1 -> R_n&e/1, Delay/1
  Sensor_data2/1 -> Bus Selector/1
  Bus Selector/1 -> Delay/2  "<QGC_sensor_reinit>"
  Bus Selector/2 -> Mux/1  "<pos_N_gps>"
  Bus Selector/3 -> Mux/2  "<pos_E_gps>"
  Mux/1 -> Delay/3
  Delay/1 -> Sum/2

== system main_RI_LIEKF/State estimation/distribute CF/Translation_estimate/Rxy_Horizontal_estimation/Rxy_kalman filter2 ==
  X : Inport
  Z : Inport  Port=2
  Enable : Inport  Port=3
  Constant : Constant  Value=F  OutDataTypeStr=single
  Constant1 : Constant  Value=Q  OutDataTypeStr=single
  Constant2 : Constant  Value=R  OutDataTypeStr=single
  Constant3 : Constant  Value=P0  OutDataTypeStr=single
  Constant4 : Constant  Value=H  OutDataTypeStr=single
  Vxy kalman filter : Subsystem  TreatAsAtomicUnit=on
  XOut : Outport
  wires:
  Enable/1 -> Vxy kalman filter/9(Enable)
  Vxy kalman filter/1(XOut) -> XOut/1
  Constant1/1 -> Vxy kalman filter/5(Q)
  Constant4/1 -> Vxy kalman filter/4(H)
  Constant2/1 -> Vxy kalman filter/6(R)
  Constant3/1 -> Vxy kalman filter/8(P0)
  Z/1 -> Vxy kalman filter/1(Z)
  Constant/1 -> Vxy kalman filter/3(G), Vxy kalman filter/2(F)
  X/1 -> Vxy kalman filter/7(X)

== system main_RI_LIEKF/State estimation/distribute CF/Translation_estimate/V_Horizontal_estimation/Integrator_V_Horizontal ==
  An : Inport
  dv : Inport  Port=2
  Sensor_data2 : Inport  Port=3
  Bus Selector : BusSelector  OutputSignals=QGC_sensor_reinit,GPS_Data.vn_gps,GPS_Data.ve_gps
  Delay : Delay  DelayLength=1  InitialConditionSource=Input port  ExternalReset=Rising
      settings: InputPortMap=u0,r5,p4
  Gain : Gain
  Gain2 : Gain  Gain=dt  SaturateOnIntegerOverflow=on  OutDataTypeStr=Inherit: Same as input  ParamDataTypeStr=Inherit: Same as input
  Mux : Mux  Inputs=2
  Scope : Scope
  Sum : Sum  Inputs=|++-
  V_n&e : Outport
  wires:
  Gain/1 -> Sum/3, Scope/1
  dv/1 -> Gain/1
  Delay/1 -> Sum/2
  Mux/1 -> Delay/3
  Bus Selector/3 -> Mux/2  "<ve_gps>"
  Bus Selector/2 -> Mux/1  "<vn_gps>"
  Bus Selector/1 -> Delay/2  "<QGC_sensor_reinit>"
  Sensor_data2/1 -> Bus Selector/1
  Sum/1 -> Delay/1, V_n&e/1
  Gain2/1 -> Sum/1
  An/1 -> Gain2/1

== system main_RI_LIEKF/State estimation/distribute CF/Translation_estimate/V_Horizontal_estimation/Rxy_kalman filter1 ==
  X : Inport
  Z : Inport  Port=2
  Enable : Inport  Port=3
  Constant : Constant  Value=F  OutDataTypeStr=single
  Constant1 : Constant  Value=Q  OutDataTypeStr=single
  Constant2 : Constant  Value=R  OutDataTypeStr=single
  Constant3 : Constant  Value=P0  OutDataTypeStr=single
  Constant4 : Constant  Value=H  OutDataTypeStr=single
  Vxy kalman filter : Subsystem  TreatAsAtomicUnit=on
  XOut : Outport
  wires:
  X/1 -> Vxy kalman filter/7(X)
  Constant/1 -> Vxy kalman filter/2(F), Vxy kalman filter/3(G)
  Z/1 -> Vxy kalman filter/1(Z)
  Constant3/1 -> Vxy kalman filter/8(P0)
  Constant2/1 -> Vxy kalman filter/6(R)
  Constant4/1 -> Vxy kalman filter/4(H)
  Constant1/1 -> Vxy kalman filter/5(Q)
  Vxy kalman filter/1(XOut) -> XOut/1
  Enable/1 -> Vxy kalman filter/9(Enable)

== system main_RI_LIEKF/State estimation/distribute CF/distribute CF/AHRS1/Bus_Constructor ==
  RF_Data : Inport
  att_quat : Inport  Port=2
  DCM_OB : Inport  Port=3
  bias_g : Inport  Port=4
  Sensor_Data : Inport  Port=5
  Bus Creator : BusCreator  Inputs=12
  Bus Selector : BusSelector  OutputSignals=IMU_Data.gyr_B_radPs,IMU_Data.acc_B_mPs2
  Bus Selector1 : BusSelector  OutputSignals=att_reset
  Bus Selector2 : BusSelector  OutputSignals=standstill
  Euler_Angle : Subsystem
  Math Function : Math  Operator=transpose  SignedPower=on
  Psi To DCM : FMT_Model_Lib/Transformation/Psi To DCM
  Signal Conversion{,1..4} (5 alike) : SignalConversion  OverrideOpt=off
  Rotation_Data : Outport
  wires:
  Bus Selector1/1 -> Signal Conversion4/1  "<att_reset>"
  Signal Conversion/1 -> Bus Creator/11  "acc_B_mPs2"
  Euler_Angle/1(phi_rad) -> Bus Creator/2  "phi_rad"
  Euler_Angle/2(theta_rad) -> Bus Creator/3  "theta_rad"
  Euler_Angle/3(psi_rad) -> Psi To DCM/1, Bus Creator/4  "psi_rad"
  Sensor_Data/1 -> Bus Selector/1
  Bus Selector2/1 -> Signal Conversion1/1  "<standstill>"
  Bus Creator/1 -> Rotation_Data/1
  bias_g/1 -> Signal Conversion3/1
  Math Function/1 -> Bus Creator/7  "M_BO"
  DCM_OB/1 -> Math Function/1, Bus Creator/8  "M_OB"
  att_quat/1 -> Euler_Angle/1(att_quat), Bus Creator/6  "att_quat"
  Psi To DCM/1 -> Bus Creator/5  "M_CO"
  Signal Conversion1/1 -> Bus Creator/12  "standstill"
  Bus Selector/2 -> Signal Conversion/1  "<acc_B_mPs2>"
  Signal Conversion2/1 -> Bus Creator/10  "gyr_B_radPs"
  Signal Conversion3/1 -> Bus Creator/9  "bias_g"
  RF_Data/1 -> Bus Selector2/1, Bus Selector1/1  "att_reset"
  Bus Selector/1 -> Signal Conversion2/1  "<gyr_B_radPs>"
  Signal Conversion4/1 -> Bus Creator/1  "att_reset"

== system main_RI_LIEKF/State estimation/distribute CF/distribute CF/AHRS1/Correct ==
  Rotation_Data : Inport
  Sensor_Data : Inport  Port=2
  RF_Data : Inport  Port=3
  Attitude_Correction : Subsystem
  Bus Selector : BusSelector  OutputSignals=standstill
  Bus Selector1 : BusSelector  OutputSignals=IMU_Data
  Gyro_Bias_Correction : Subsystem
  att_B_correction : Outport
  bias_g_B_correction : Outport  Port=2
  wires:
  Gyro_Bias_Correction/1(bias_g_B_correction) -> bias_g_B_correction/1
  Bus Selector1/1 -> Gyro_Bias_Correction/2(IMU_Data)  "<IMU_Data>"
  RF_Data/1 -> Bus Selector/1
  Attitude_Correction/1(att_B_correction) -> att_B_correction/1, Gyro_Bias_Correction/1(att_B_correction)
  Sensor_Data/1 -> Attitude_Correction/1(Sensor_Data), Bus Selector1/1
  Rotation_Data/1 -> Attitude_Correction/2(Rotation_Data)
  Bus Selector/1 -> Attitude_Correction/3(standstill)  "<standstill>"

== system main_RI_LIEKF/State estimation/distribute CF/distribute CF/AHRS1/Update ==
  att_B_correction : Inport
  bias_g_correction : Inport  Port=2
  RF_Data : Inport  Port=3
  Sensor_Data : Inport  Port=4
  Attitude_Update : Subsystem
  Bus Selector : BusSelector  OutputSignals=IMU_Data.gyr_B_radPs
  Bus Selector1 : BusSelector  OutputSignals=att_reset,quat_0
  Gyro_Bias_Update : Subsystem
  Sum2 : Sum  Inputs=|++
  att_quat : Outport
  DCM_OB : Outport  Port=2
  bias_g : Outport  Port=3
  wires:
  Sensor_Data/1 -> Bus Selector/1
  Gyro_Bias_Update/1(gyr_B_correction) -> Sum2/2
  att_B_correction/1 -> Sum2/1
  Sum2/1 -> Attitude_Update/3(att_B_correction)
  Bus Selector/1 -> Gyro_Bias_Update/2(gyr_B_radPs)  "<gyr_B_radPs>"
  bias_g_correction/1 -> Gyro_Bias_Update/1(bias_g_correction)
  Attitude_Update/1(att_quat) -> att_quat/1
  Attitude_Update/2(DCM_OB) -> DCM_OB/1
  Gyro_Bias_Update/2(bias_g) -> bias_g/1
  RF_Data/1 -> Bus Selector1/1  "att_reset"
  Bus Selector1/1 -> Attitude_Update/1(att_reset)  "<att_reset>"
  Bus Selector1/2 -> Attitude_Update/2(quat_0)  "<quat_0>"

== system main_RI_LIEKF/State estimation/distribute CF/distribute CF/Bus_Constructor/Euler_Angle ==
  att_quat : Inport
  Demux : Demux  Outputs=3
  Quaternions to Rotation Angles : sharedtransform/Quaternions to Rotation Angles  rotationOrder=ZYX  aMode=aMode
  phi_rad : Outport
  theta_rad : Outport  Port=2
  psi_rad : Outport  Port=3
  wires:
  Demux/1 -> phi_rad/1
  Demux/2 -> theta_rad/1
  Demux/3 -> psi_rad/1
  att_quat/1 -> Quaternions to Rotation Angles/1
  Quaternions to Rotation Angles/1 -> Demux/1

== system main_RI_LIEKF/State estimation/distribute CF/distribute CF/Bus_Constructor/Subsystem1 ==
  psi : Inport
  Gain : Gain  Gain=-1
  Subsystem : Subsystem
  DCMz : Outport
  wires:
  psi/1 -> Gain/1
  Gain/1 -> Subsystem/1(psi)
  Subsystem/1(DCMz) -> DCMz/1

== system main_RI_LIEKF/State estimation/distribute CF/distribute CF/Correct/Attitude_Correction ==
  note: N系到B系
  Sensor_Data : Inport
  Rotation_Data : Inport  Port=2
  Attitude_Correct : Subsystem
  Bus Selector2 : BusSelector  OutputSignals=M_BO
  Mag_Correct : Subsystem
  Multiply : Product  Multiplication=Matrix(*)
  Scope : Scope
  Sum : Sum  Inputs=|++
  att_B_correction : Outport
  wires:
  Multiply/1 -> att_B_correction/1
  Rotation_Data/1 -> Bus Selector2/1, Attitude_Correct/2(Rotation_Data), Mag_Correct/1(Rotation_Data)
  Sensor_Data/1 -> Mag_Correct/2(Sensor_Data), Attitude_Correct/1(Sensor_Data)
  Bus Selector2/1 -> Multiply/1  "<M_BO>"
  Sum/1 -> Multiply/2
  Attitude_Correct/1(att_corr_O) -> Sum/1
  Mag_Correct/1(mag_corr_O) -> Scope/1  "mag_corr_O"

== system main_RI_LIEKF/State estimation/distribute CF/distribute CF/Correct/Subsystem2 ==
  note: 零速判断
  note: 误差角r
  note: 误差角速度r‘
  Sensor_Data : Inport
  att_B_correction : Inport  Port=2
  Abs : Abs  SaturateOnIntegerOverflow=off
  Bus Selector1 : BusSelector  OutputSignals=IMU_Data.accl_B_m/s2_LPF
  Compare To Constant : simulink/Logic and Bit Operations/Compare To Constant  relop=<=  const=1  OutDataTypeStr=boolean
  Constant : Constant  Value=g0  OutDataTypeStr=single
  Data Type Conversion : DataTypeConversion  OutDataTypeStr=single  SaturateOnIntegerOverflow=off  RndMeth=Floor
  Gain1 : Gain  Gain=gbias_correct_gain
  MX Product1 : Product  RndMeth=Simplest
  Saturation2 : Saturate  UpperLimit=0.1/180*pi  LowerLimit=-0.1/180*pi
  Scope : Scope
  Scope1 : Scope  NumInputPorts=2
  Subtract : Sum  Inputs=+-
  norm : Subsystem
  低通滤波 : Subsystem  mask{fc=5, zeta=0.707}
      mask prompts: fc "Cut-off frequence"; zeta "Damping factor"
      mask DialogControl ParameterGroupVar Prompt: 参数
  bias_g_B_correction : Outport
  wires:
  Sensor_Data/1 -> Bus Selector1/1
  Saturation2/1 -> bias_g_B_correction/1  "bias_g_correction"
  Constant/1 -> Subtract/2
  Compare To Constant/1 -> Data Type Conversion/1
  att_B_correction/1 -> MX Product1/1
  Data Type Conversion/1 -> Scope/1, MX Product1/2
  MX Product1/1 -> Scope1/1, 低通滤波/1(u)
  Subtract/1 -> Abs/1
  norm/1(Out1) -> Subtract/1
  Bus Selector1/1 -> norm/1(In1)  "<accl_B_m/s2_LPF>"
  Abs/1 -> Compare To Constant/1
  Gain1/1 -> Saturation2/1
  低通滤波/1(y) -> Scope1/2, Gain1/1

== system main_RI_LIEKF/State estimation/distribute CF/distribute CF/Translation_estimate/Rxy_Horizontal_estimation ==
  Vn : Inport
  Enable : Inport  Port=2
  Sensor_data2 : Inport  Port=3
  Cbn : Inport  Port=4
  Add1 : Sum  Inputs=+-
  Bus Selector1 : BusSelector  OutputSignals=GPS_Data.pos_N_gps,GPS_Data.pos_E_gps
  Data Store Memory : DataStoreMemory  DataStoreName=GPS_enable_CF  WriteAfterWriteMsg=warning  ShowAdditionalParam=off
  Data Store Read : DataStoreRead  DataStoreName=GPS_enable_CF  IndexOptions=Index vector (dialog)  Indices=1  OutputSizes=1
  Data Store Write : DataStoreWrite  DataStoreName=GPS_enable_CF  IndexOptions=Index vector (dialog)  Indices=1  OutputSizes=1
  Delay1 : Delay  DelayLength=1
  Integrator_R_Horizontal : Subsystem
  Mux1 : Mux  Inputs=2
  Rxy_kalman filter2 : Subsystem  mask{F=diag([-0.1,-0.1,-0.01,-0.01]), H=[1,0,-1,0;0,1,0,-1], Q=diag([1,1,0.1,0.1]), R=diag([0.05,0.05]), P0=diag([0.8,0.8,0.2,0.2])}
      mask prompts: F "状态转移矩阵：F"; H "观测转移矩阵：H"; Q "预测噪声协方差矩阵：Q"; R "量测噪声协方差矩阵：R"; P0 "初始协方差矩阵：P0"
      mask DialogControl DescTextVar Prompt: Kalman Filter
  Scope : Scope
  Scope1 : Scope  NumInputPorts=2
  Scope5 : Scope
  Selector1 : Selector  InputPortWidth=4  IndexOptions=Index vector (dialog)  Indices=[1 2]  OutputSizes=1
  Subsystem : Subsystem
  R_n&e : Outport
  wires:
  Vn/1 -> Integrator_R_Horizontal/1(Vn)
  Add1/1 -> Rxy_kalman filter2/2(Z)
  Rxy_kalman filter2/1(XOut) -> Scope/1, Delay1/1
  Bus Selector1/1 -> Mux1/1  "<pos_N_gps>"
  Integrator_R_Horizontal/1(R_n&e) -> R_n&e/1
  Bus Selector1/2 -> Mux1/2  "<pos_E_gps>"
  Sensor_data2/1 -> Bus Selector1/1, Integrator_R_Horizontal/3(Sensor_data2)
  Delay1/1 -> Rxy_kalman filter2/1(X), Selector1/1
  Mux1/1 -> Scope1/2, Add1/2
  Selector1/1 -> Integrator_R_Horizontal/2(dR)
  Cbn/1 -> Integrator_R_Horizontal/4(Cbn)
  Integrator_R_Horizontal/2(R_n&eL) -> Scope1/1, Add1/1
  Subsystem/1(flag) -> Scope5/1, Data Store Write/1
  Data Store Read/1 -> Rxy_kalman filter2/3(Enable)

== system main_RI_LIEKF/State estimation/distribute CF/distribute CF/Translation_estimate/V_Horizontal_estimation ==
  note: 0530改：
      | 加入GPStype限制
  An : Inport
  Sensor_data2 : Inport  Port=2
  Add : Sum  Inputs=+-
  Bus Selector2 : BusSelector  OutputSignals=GPS_Data.vn_gps,GPS_Data.ve_gps,GPS_Data.fixtype_gps
  Compare To Constant : simulink/Logic and Bit Operations/Compare To Constant  relop=>=  const=1  OutDataTypeStr=boolean
  Delay : Delay  DelayLength=1
  Detect Change : simulink/Logic and Bit Operations/Detect Change  vinit=0  OutDataTypeStr=boolean
  Integrator_V_Horizontal : Subsystem
  Logical Operator : Logic  AllPortsSameDT=off  OutDataTypeStr=boolean
  Mux : Mux  Inputs=2
  Rxy_kalman filter1 : Subsystem  mask{F=diag([-0.1,-0.1,-0.01,-0.01]), H=[1,0,-1,0;0,1,0,-1], Q=diag([1,1,0.1,0.1]), R=diag([0.1,0.1]), P0=diag([0.8,0.8,0.5,0.5])}
      mask prompts: F "状态转移矩阵：F"; H "观测转移矩阵：H"; Q "预测噪声协方差矩阵：Q"; R "量测噪声协方差矩阵：R"; P0 "初始协方差矩阵：P0"
      mask DialogControl DescTextVar Prompt: Kalman Filter
  Scope : Scope  NumInputPorts=2
  Scope1 : Scope
  Selector : Selector  InputPortWidth=4  IndexOptions=Index vector (dialog)  Indices=[1 2]  OutputSizes=1
  vxy_estimout : Outport
  V_n&e : Outport  Port=2
  GPS_v_enable : Outport  Port=3
  wires:
  Logical Operator/1 -> Rxy_kalman filter1/3(Enable), GPS_v_enable/1, Scope1/1
  Compare To Constant/1 -> Logical Operator/2
  Detect Change/1 -> Logical Operator/1
  Bus Selector2/3 -> Compare To Constant/1  "<fixtype_gps>"
  Sensor_data2/1 -> Integrator_V_Horizontal/3(Sensor_data2), Bus Selector2/1
  An/1 -> Integrator_V_Horizontal/1(An)
  Add/1 -> Rxy_kalman filter1/2(Z)
  Integrator_V_Horizontal/1(V_n&e) -> Add/1, Scope/1, vxy_estimout/1, V_n&e/1
  Rxy_kalman filter1/1(XOut) -> Delay/1
  Bus Selector2/2 -> Mux/2  "<ve_gps>"
  Mux/1 -> Add/2, Scope/2
  Bus Selector2/1 -> Detect Change/1, Mux/1  "<vn_gps>"
  Selector/1 -> Integrator_V_Horizontal/2(dv)
  Delay/1 -> Rxy_kalman filter1/1(X), Selector/1

== system main_RI_LIEKF/State estimation/distribute CF/distribute CF/Translation_estimate/translate to N ==
  RotationData : Inport
  Sensor_data : Inport  Port=2
  Bus Selector2 : BusSelector  OutputSignals=IMU_Data.accl_B_m/s2_LPF
  Bus Selector3 : BusSelector  OutputSignals=M_OB
  Product : Product  Multiplication=Matrix(*)
  Selector : Selector  InputPortWidth=3  IndexOptions=Index vector (dialog)  Indices=[1 2]  OutputSizes=1
  Selector1 : Selector  InputPortWidth=3  IndexOptions=Index vector (dialog)  Indices=[3]  OutputSizes=1
  accel_Horizontal_predict : Outport
  accel_Vertical_predict : Outport  Port=2
  wires:
  Selector1/1 -> accel_Vertical_predict/1
  Selector/1 -> accel_Horizontal_predict/1
  Product/1 -> Selector/1, Selector1/1
  Sensor_data/1 -> Bus Selector2/1
  Bus Selector3/1 -> Product/1  "<M_OB>"
  Bus Selector2/1 -> Product/2  "<accl_B_m/s2_LPF>"
  RotationData/1 -> Bus Selector3/1
